simulink model "gm_pwm_generator"  (R2024b)
settings: Solver=FixedStepDiscrete  StartTime=0.0  StopTime=2  FixedStep=1e-06  RelTol=1e-3
settings Model: Creator=jpimentel3  LastModifiedBy=jpimentel3
settings OptimizationCC: BlockReduction=off  ConditionallyExecuteInputs=off  DefaultParameterBehavior=Inlined
settings DebuggingCC: AlgebraicLoopMsg=error  InheritedTsInSrcMsg=none
settings HardwareCC: ProdBitPerPointer=32  ProdBitPerSizeT=32  ProdBitPerPtrDiffT=32  ProdLargestAtomicFloat=None  ProdIntDivRoundTo=Undefined  ProdEndianess=Unspecified  ProdWordSize=32  ProdHWDeviceType=ASIC/FPGA->ASIC/FPGA  TargetBitPerPointer=64  TargetBitPerSizeT=64  TargetBitPerPtrDiffT=64  TargetLongLongMode=on  TargetIntDivRoundTo=Zero  TargetEndianess=LittleEndian  TargetWordSize=64  TargetHWDeviceType=Custom Processor->MATLAB Host Computer  ProdEqTarget=off

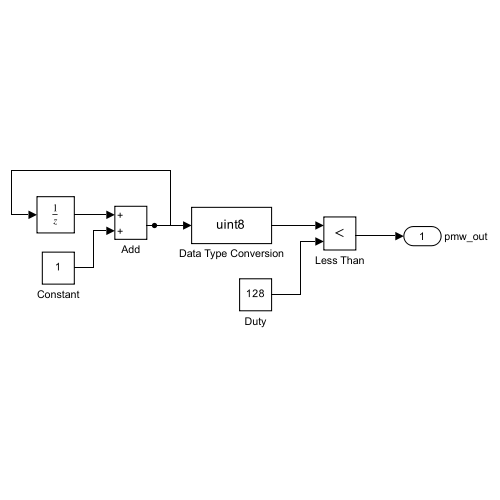
[thumbnail: Simulink's stored preview of the top-level diagram]
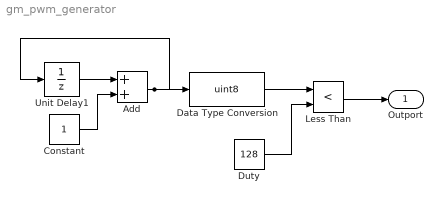
== system gm_pwm_generator ==
  Add : Sum  OutMax=255  OutDataTypeStr=uint8
  Constant : Constant  OutDataTypeStr=uint8
  Data Type Conversion : DataTypeConversion  OutMin=0  OutMax=255  OutDataTypeStr=uint8  SaturateOnIntegerOverflow=off  RndMeth=Floor
  Duty : Constant  Value=128  OutDataTypeStr=uint8
  Less Than : RelationalOperator  Operator=<  OutDataTypeStr=boolean  RndMeth=Simplest  InputSameDT=off
  Unit Delay1 : UnitDelay  SampleTime=-1  HasFrameUpgradeWarning=on
  Outport : Outport  SignalName=pmw_out  SampleTime=1e-06
  wires:
  Constant/1 -> Add/2
  Unit Delay1/1 -> Add/1
  Add/1 -> Unit Delay1/1, Data Type Conversion/1
  Data Type Conversion/1 -> Less Than/1
  Duty/1 -> Less Than/2
  Less Than/1 -> Outport/1
